simulink model "drone_dynamics"  (R2026a)
settings: Solver=VariableStepAuto  StopTime=500e-3  FixedStep=1e-3  MaxStep=5e-6  MinStep=1e-7
undefined symbols (not defined in the file): b, J, K_Q, K_t, K_w, L, P, R, Vpp
libraries: simulink x2
settings Model: Creator=codykremer  LastModifiedBy=codykremer

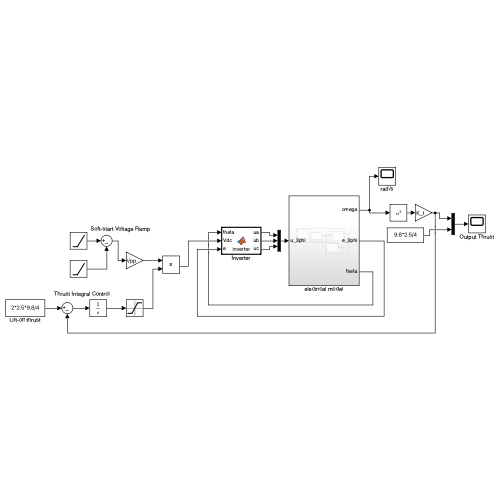
[thumbnail: Simulink's stored preview of the top-level diagram]
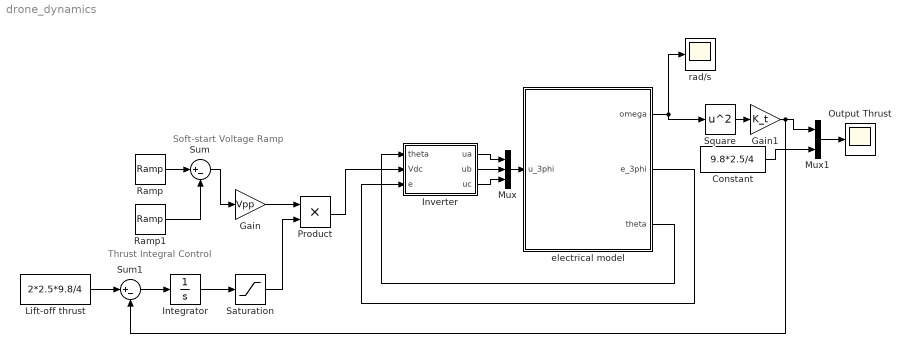
== system drone_dynamics ==
  note: Soft-start Voltage Ramp
  note: Thrust Integral Control
  Constant : Constant  Value=9.8*2.5/4
  Gain : Gain  Gain=Vpp
  Gain1 : Gain  Gain=K_t
  Integrator : Integrator
  Inverter : MATLAB Function  TreatAsAtomicUnit=on
  Lift-off thrust : Constant  Value=2*2.5*9.8/4
  Mux : Mux  Inputs=3
  Mux1 : Mux  Inputs=2
  Output Thrust : Scope
      settings: ActiveDisplayYMinimum=-1.891050775571288  ActiveDisplayYMaximum=17.019456980141594  DataLoggingVariableName=ScopeData3
  Product : Product
  Ramp : simulink/Sources/Ramp  slope=1/0.1  start=0  InitialOutput=0
  Ramp1 : simulink/Sources/Ramp  slope=1/0.1  start=0.1  InitialOutput=0
  Saturation : Saturate  UpperLimit=1  LowerLimit=0
  Square : Math  Operator=square
  Sum : Sum  Inputs=|+-
  Sum1 : Sum  Inputs=|+-
  electrical model : Subsystem
  rad/s : Scope
      settings: ActiveDisplayYMinimum=-264.86771140334332  ActiveDisplayYMaximum=2383.8094026300905  DataLoggingVariableName=ScopeData9
  wires:
  electrical model/1(omega) -> rad/s/1, Square/1
  Inverter/1(ua) -> Mux/1
  Inverter/3(uc) -> Mux/3
  Inverter/2(ub) -> Mux/2
  Mux/1 -> electrical model/1(u_3phi)
  electrical model/3(theta) -> Inverter/1(theta)
  electrical model/2(e_3phi) -> Inverter/3(e)
  Ramp/1 -> Sum/1
  Ramp1/1 -> Sum/2
  Sum/1 -> Gain/1
  Square/1 -> Gain1/1
  Gain1/1 -> Sum1/2, Mux1/1
  Constant/1 -> Mux1/2
  Mux1/1 -> Output Thrust/1
  Lift-off thrust/1 -> Sum1/1
  Gain/1 -> Product/1
  Product/1 -> Inverter/2(Vdc)
  Saturation/1 -> Product/2
  Integrator/1 -> Saturation/1
  Sum1/1 -> Integrator/1

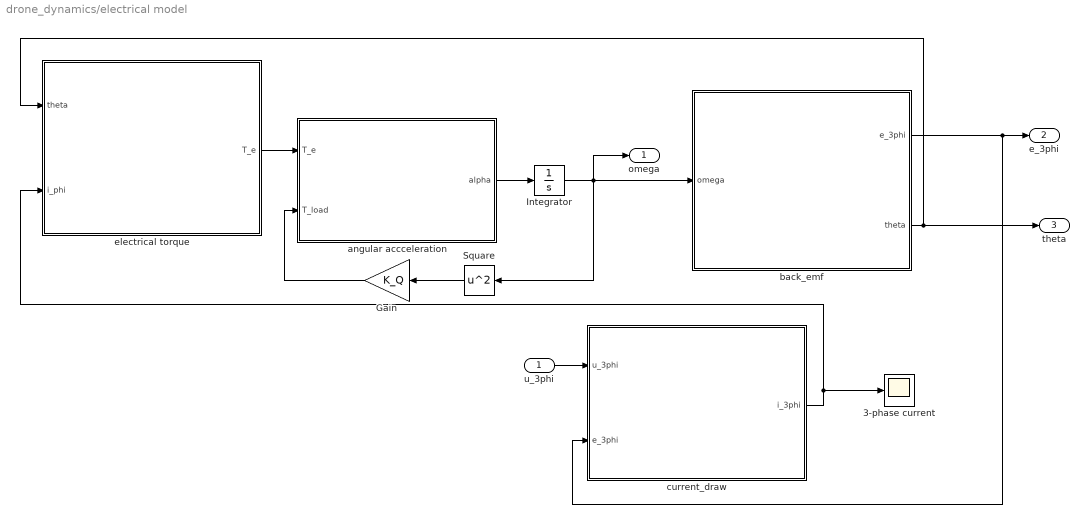
== system drone_dynamics/electrical model ==
  u_3phi : Inport
  "3-phase current " : Scope
      settings: ActiveDisplayYMinimum=-26.947199074387367  ActiveDisplayYMaximum=26.8640591960215  DataLoggingVariableName=ScopeData2
  Gain : Gain  Gain=K_Q
  Integrator : Integrator
  Square : Math  Operator=square
  angular accceleration : Subsystem
  back_emf : Subsystem
  current_draw : Subsystem
  electrical torque : Subsystem
  omega : Outport
  e_3phi : Outport  Port=2
  theta : Outport  Port=3
  wires:
  angular accceleration/1(alpha) -> Integrator/1
  back_emf/1(e_3phi) -> e_3phi/1, current_draw/2(e_3phi)
  current_draw/1(i_3phi) -> electrical torque/2(i_phi), "3-phase current "/1
  Integrator/1 -> Square/1, omega/1, back_emf/1(omega)
  electrical torque/1(T_e) -> angular accceleration/1(T_e)
  Square/1 -> Gain/1
  u_3phi/1 -> current_draw/1(u_3phi)
  back_emf/2(theta) -> theta/1, electrical torque/1(theta)
  Gain/1 -> angular accceleration/2(T_load)

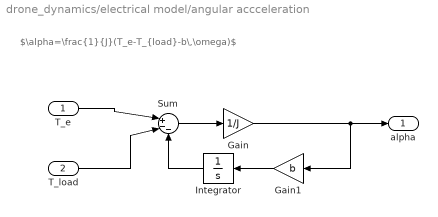
== system drone_dynamics/electrical model/angular accceleration ==
  note: $\alpha=\frac{1}{J}(T_e-T_{load}-b\,\omega)$
  T_e : Inport
  T_load : Inport  Port=2
  Gain : Gain  Gain=1/J
  Gain1 : Gain  Gain=b
  Integrator : Integrator
  Sum : Sum  Inputs=|+--
  alpha : Outport
  wires:
  Gain/1 -> Gain1/1, alpha/1
  T_e/1 -> Sum/1
  T_load/1 -> Sum/2
  Sum/1 -> Gain/1
  Integrator/1 -> Sum/3
  Gain1/1 -> Integrator/1

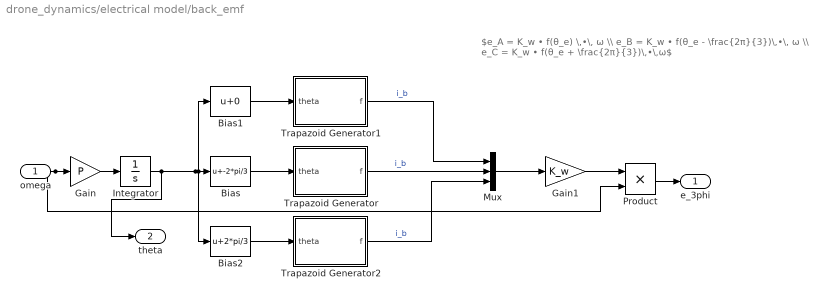
== system drone_dynamics/electrical model/back_emf ==
  note: $e_A = K_w • f(θ_e) \,•\, ω \\ e_B = K_w • f(θ_e - \frac{2π}{3})\,•\, ω \\ e_C = K_w • f(θ_e + \frac{2π}{3})\,•\,ω$
  omega : Inport
  Bias : Bias  Bias=-2*pi/3  SaturateOnIntegerOverflow=off
  Bias1 : Bias  SaturateOnIntegerOverflow=off
  Bias2 : Bias  Bias=2*pi/3  SaturateOnIntegerOverflow=off
  Gain : Gain  Gain=P
  Gain1 : Gain  Gain=K_w
  Integrator : Integrator
  Mux : Mux  Inputs=3
  Product : Product
  Trapazoid Generator : MATLAB Function  TreatAsAtomicUnit=on
  Trapazoid Generator1 : MATLAB Function  TreatAsAtomicUnit=on
  Trapazoid Generator2 : MATLAB Function  TreatAsAtomicUnit=on
  e_3phi : Outport
  theta : Outport  Port=2
  wires:
  Bias/1 -> Trapazoid Generator/1(theta)
  Gain/1 -> Integrator/1
  Integrator/1 -> theta/1, Bias1/1, Bias2/1, Bias/1
  Trapazoid Generator/1(f) -> Mux/2  "i_b"
  omega/1 -> Product/2, Gain/1
  Bias1/1 -> Trapazoid Generator1/1(theta)
  Trapazoid Generator2/1(f) -> Mux/3  "i_b"
  Bias2/1 -> Trapazoid Generator2/1(theta)
  Trapazoid Generator1/1(f) -> Mux/1  "i_b"
  Mux/1 -> Gain1/1
  Product/1 -> e_3phi/1
  Gain1/1 -> Product/1

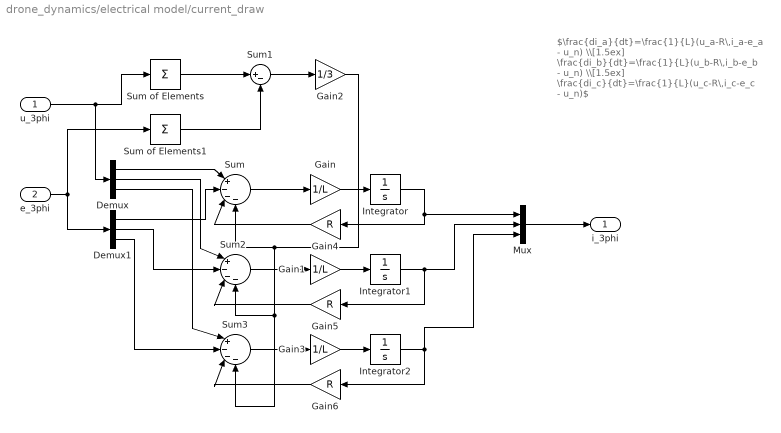
== system drone_dynamics/electrical model/current_draw ==
  note: $\frac{di_a}{dt}=\frac{1}{L}(u_a-R\,i_a-e_a - u_n) \\[1.5ex] \frac{di_b}{dt}=\frac{1}{L}(u_b-R\,i_b-e_b - u_n) \\[1.5ex] \frac{di_c}{dt}=\frac{1}{L}(u_c-R\,i_c-e_c - u_n)$
  u_3phi : Inport
  e_3phi : Inport  Port=2
  Demux : Demux  Outputs=3
  Demux1 : Demux  Outputs=3
  Gain : Gain  Gain=1/L
  Gain1 : Gain  Gain=1/L
  Gain2 : Gain  Gain=1/3
  Gain3 : Gain  Gain=1/L
  Gain4 : Gain  Gain=R
  Gain5 : Gain  Gain=R
  Gain6 : Gain  Gain=R
  Integrator : Integrator
  Integrator1 : Integrator
  Integrator2 : Integrator
  Mux : Mux  Inputs=3
  Sum : Sum  Inputs=|+---
  Sum of Elements : Sum  Inputs=+
  Sum of Elements1 : Sum  Inputs=+
  Sum1 : Sum  Inputs=|+-
  Sum2 : Sum  Inputs=|+---
  Sum3 : Sum  Inputs=|+---
  i_3phi : Outport
  wires:
  u_3phi/1 -> Demux/1, Sum of Elements/1
  e_3phi/1 -> Demux1/1, Sum of Elements1/1
  Sum1/1 -> Gain2/1
  Sum of Elements/1 -> Sum1/1
  Sum of Elements1/1 -> Sum1/2
  Mux/1 -> i_3phi/1
  Demux/1 -> Sum/1
  Demux/2 -> Sum2/1
  Demux/3 -> Sum3/1
  Demux1/1 -> Sum/2
  Demux1/2 -> Sum2/2
  Demux1/3 -> Sum3/2
  Sum/1 -> Gain/1
  Sum2/1 -> Gain1/1
  Sum3/1 -> Gain3/1
  Gain/1 -> Integrator/1
  Gain1/1 -> Integrator1/1
  Gain3/1 -> Integrator2/1
  Integrator/1 -> Gain4/1, Mux/1
  Integrator1/1 -> Mux/2, Gain5/1
  Integrator2/1 -> Mux/3, Gain6/1
  Gain6/1 -> Sum3/3
  Gain5/1 -> Sum2/3
  Gain4/1 -> Sum/3
  Gain2/1 -> Sum/4, Sum3/4, Sum2/4

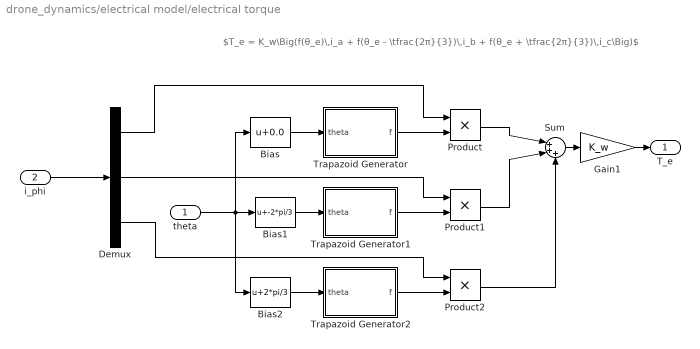
== system drone_dynamics/electrical model/electrical torque ==
  note: $T_e = K_w\Big(f(θ_e)\,i_a + f(θ_e - \tfrac{2π}{3})\,i_b + f(θ_e + \tfrac{2π}{3})\,i_c\Big)$
  theta : Inport
  i_phi : Inport  Port=2
  Bias : Bias  Bias=0.0  SaturateOnIntegerOverflow=off
  Bias1 : Bias  Bias=-2*pi/3  SaturateOnIntegerOverflow=off
  Bias2 : Bias  Bias=2*pi/3  SaturateOnIntegerOverflow=off
  Demux : Demux  Outputs=3
  Gain1 : Gain  Gain=K_w
  Product : Product
  Product1 : Product
  Product2 : Product
  Sum : Sum  Inputs=|+++
  Trapazoid Generator : MATLAB Function  TreatAsAtomicUnit=on
  Trapazoid Generator1 : MATLAB Function  TreatAsAtomicUnit=on
  Trapazoid Generator2 : MATLAB Function  TreatAsAtomicUnit=on
  T_e : Outport
  wires:
  Demux/1 -> Product/1
  Trapazoid Generator1/1(f) -> Product1/2
  Product1/1 -> Sum/2
  Product2/1 -> Sum/3
  Trapazoid Generator/1(f) -> Product/2
  Trapazoid Generator2/1(f) -> Product2/2
  Demux/3 -> Product2/1
  Sum/1 -> Gain1/1
  Gain1/1 -> T_e/1
  Product/1 -> Sum/1
  Demux/2 -> Product1/1
  i_phi/1 -> Demux/1
  Bias/1 -> Trapazoid Generator/1(theta)
  Bias1/1 -> Trapazoid Generator1/1(theta)
  Bias2/1 -> Trapazoid Generator2/1(theta)
  theta/1 -> Bias/1, Bias2/1, Bias1/1

== matlab function drone_dynamics/electrical model/electrical torque/Trapazoid Generator ==
  data: theta input; f output
function f = trapezoidal_shape(theta)
%TRAPEZOIDAL_SHAPE  Vectorized normalized trapezoidal BEMF shape function.
%   Returns f in [-1, 1]: 120-degree flat top/bottom regions separated by
%   60-degree linear transitions, period 2*pi. Used as
%   e = K_w * f(theta_e) * omega.

    phi = mod(theta + pi/6, 2*pi);
    f = -ones(size(phi));                     % default: flat bottom

    idx1 = phi < pi/3;
    f(idx1) = -1 + (6/pi)*phi(idx1);          % rising ramp

    idx2 = (phi >= pi/3) & (phi < pi);
    f(idx2) = 1;                              % flat top

    idx3 = (phi >= pi) & (phi < 4*pi/3);
    f(idx3) = 1 - (6/pi)*(phi(idx3) - pi);    % falling ramp
    % remaining elements (phi >= 4*pi/3) stay at -1, already set above
end

== matlab function drone_dynamics/electrical model/electrical torque/Trapazoid Generator1 ==
  data: theta input; f output
function f = trapezoidal_shape(theta)
%TRAPEZOIDAL_SHAPE  Vectorized normalized trapezoidal BEMF shape function.
%   Returns f in [-1, 1]: 120-degree flat top/bottom regions separated by
%   60-degree linear transitions, period 2*pi. Used as
%   e = K_w * f(theta_e) * omega.

    phi = mod(theta + pi/6, 2*pi);
    f = -ones(size(phi));                     % default: flat bottom

    idx1 = phi < pi/3;
    f(idx1) = -1 + (6/pi)*phi(idx1);          % rising ramp

    idx2 = (phi >= pi/3) & (phi < pi);
    f(idx2) = 1;                              % flat top

    idx3 = (phi >= pi) & (phi < 4*pi/3);
    f(idx3) = 1 - (6/pi)*(phi(idx3) - pi);    % falling ramp
    % remaining elements (phi >= 4*pi/3) stay at -1, already set above
end

== matlab function drone_dynamics/electrical model/electrical torque/Trapazoid Generator2 ==
  data: theta input; f output
function f = trapezoidal_shape(theta)
%TRAPEZOIDAL_SHAPE  Vectorized normalized trapezoidal BEMF shape function.
%   Returns f in [-1, 1]: 120-degree flat top/bottom regions separated by
%   60-degree linear transitions, period 2*pi. Used as
%   e = K_w * f(theta_e) * omega.

    phi = mod(theta + pi/6, 2*pi);
    f = -ones(size(phi));                     % default: flat bottom

    idx1 = phi < pi/3;
    f(idx1) = -1 + (6/pi)*phi(idx1);          % rising ramp

    idx2 = (phi >= pi/3) & (phi < pi);
    f(idx2) = 1;                              % flat top

    idx3 = (phi >= pi) & (phi < 4*pi/3);
    f(idx3) = 1 - (6/pi)*(phi(idx3) - pi);    % falling ramp
    % remaining elements (phi >= 4*pi/3) stay at -1, already set above
end

== matlab function drone_dynamics/electrical model/back_emf/Trapazoid Generator ==
  data: theta input; f output
function f = trapezoidal_shape(theta)
%TRAPEZOIDAL_SHAPE  Vectorized normalized trapezoidal BEMF shape function.
%   Returns f in [-1, 1]: 120-degree flat top/bottom regions separated by
%   60-degree linear transitions, period 2*pi. Used as
%   e = K_w * f(theta_e) * omega.

    phi = mod(theta + pi/6, 2*pi);
    f = -ones(size(phi));                     % default: flat bottom

    idx1 = phi < pi/3;
    f(idx1) = -1 + (6/pi)*phi(idx1);          % rising ramp

    idx2 = (phi >= pi/3) & (phi < pi);
    f(idx2) = 1;                              % flat top

    idx3 = (phi >= pi) & (phi < 4*pi/3);
    f(idx3) = 1 - (6/pi)*(phi(idx3) - pi);    % falling ramp
    % remaining elements (phi >= 4*pi/3) stay at -1, already set above
end

== matlab function drone_dynamics/electrical model/back_emf/Trapazoid Generator1 ==
  data: theta input; f output
function f = trapezoidal_shape(theta)
%TRAPEZOIDAL_SHAPE  Vectorized normalized trapezoidal BEMF shape function.
%   Returns f in [-1, 1]: 120-degree flat top/bottom regions separated by
%   60-degree linear transitions, period 2*pi. Used as
%   e = K_w * f(theta_e) * omega.

    phi = mod(theta + pi/6, 2*pi);
    f = -ones(size(phi));                     % default: flat bottom

    idx1 = phi < pi/3;
    f(idx1) = -1 + (6/pi)*phi(idx1);          % rising ramp

    idx2 = (phi >= pi/3) & (phi < pi);
    f(idx2) = 1;                              % flat top

    idx3 = (phi >= pi) & (phi < 4*pi/3);
    f(idx3) = 1 - (6/pi)*(phi(idx3) - pi);    % falling ramp
    % remaining elements (phi >= 4*pi/3) stay at -1, already set above
end

== matlab function drone_dynamics/electrical model/back_emf/Trapazoid Generator2 ==
  data: theta input; f output
function f = trapezoidal_shape(theta)
%TRAPEZOIDAL_SHAPE  Vectorized normalized trapezoidal BEMF shape function.
%   Returns f in [-1, 1]: 120-degree flat top/bottom regions separated by
%   60-degree linear transitions, period 2*pi. Used as
%   e = K_w * f(theta_e) * omega.

    phi = mod(theta + pi/6, 2*pi);
    f = -ones(size(phi));                     % default: flat bottom

    idx1 = phi < pi/3;
    f(idx1) = -1 + (6/pi)*phi(idx1);          % rising ramp

    idx2 = (phi >= pi/3) & (phi < pi);
    f(idx2) = 1;                              % flat top

    idx3 = (phi >= pi) & (phi < 4*pi/3);
    f(idx3) = 1 - (6/pi)*(phi(idx3) - pi);    % falling ramp
    % remaining elements (phi >= 4*pi/3) stay at -1, already set above
end

== matlab function drone_dynamics/Inverter ==
  data: theta input; ua output; Vdc input; ub output; uc output; e input

function [ua, ub, uc] = inverter(theta, Vdc, e)
arguments
    theta (1,1)
    Vdc (1,1)
    e (3,1)
end
theta = mod(theta, 2*pi);
sector = floor(theta/(2*pi/6)) + 1;
sum_e = sum(e);

ua = e(1);
ub = e(2);
uc = e(3); 

switch sector
    case 1
        ua = Vdc/2;  ub = -Vdc/2; uc = (3*e(3) - sum_e)/2;
    case 2
        ua = Vdc/2;  ub = (3*e(2) - sum_e)/2; uc = -Vdc/2;
    case 3
        ua = (3*e(1) - sum_e)/2; ub = Vdc/2;  uc = -Vdc/2;
    case 4
        ua = -Vdc/2; ub = Vdc/2;  uc = (3*e(3) - sum_e)/2;
    case 5
        ua = -Vdc/2; ub = (3*e(2) - sum_e)/2; uc = Vdc/2;
    case 6
        ua = (3*e(1) - sum_e)/2; ub = -Vdc/2; uc = Vdc/2;
end
end
